simulink model "uas_joystick"  (R2021a)
settings: Solver=VariableStepAuto  StartTime=0.0  StopTime=60  RelTol=1e-3
undefined symbols (not defined in the file or in its folder): Angular, Linear
libraries: robotlib x2, vrlib x1
settings Model: EnablePacing=on  Creator=dwuth  LastModifiedBy=dwuth

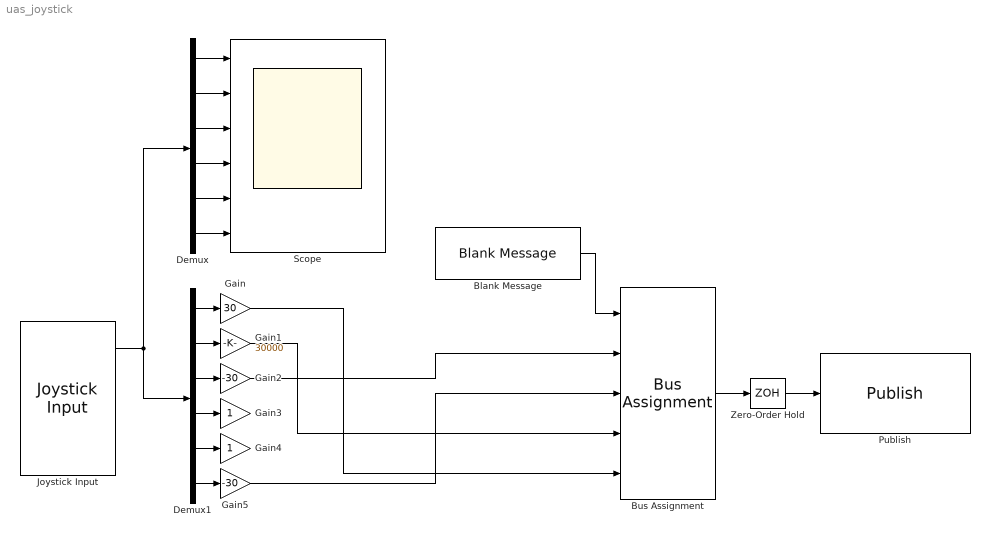
== system uas_joystick ==
  Blank Message : robotlib/Blank Message  messageClass=Message  entityType=geometry_msgs/Twist  messageType=geometry_msgs/Twist  SampleTime=inf  legacyBusStruct=off
  Bus Assignment : BusAssignment  AssignedSignals=Linear.X,Linear.Y,Linear.Z,Angular.Z
  Demux : Demux  Outputs=6
  Demux1 : Demux  Outputs=6
  Gain : Gain  Gain=30
  Gain1 : Gain  Gain=30000
  Gain2 : Gain  Gain=-30
  Gain3 : Gain
  Gain4 : Gain
  Gain5 : Gain  Gain=-30
  Joystick Input : vrlib/Joystick Input  joyid=1  adjustports=on  forcefeed=off
  Publish : robotlib/Publish  topicSource=Specify your own  topic=/crazyflie/cmd_vel  messageType=geometry_msgs/Twist  legacyBusStruct=off  messageQueueLength=1
  Scope : Scope  NumInputPorts=6
  Zero-Order Hold : ZeroOrderHold  SampleTime=25
  wires:
  Demux/1 -> Scope/1
  Demux/2 -> Scope/2
  Demux/3 -> Scope/3
  Demux/4 -> Scope/4
  Demux/5 -> Scope/5
  Demux/6 -> Scope/6
  Joystick Input/1 -> Demux1/1, Demux/1
  Demux1/1 -> Gain/1
  Demux1/2 -> Gain1/1
  Demux1/3 -> Gain2/1
  Demux1/4 -> Gain3/1
  Demux1/5 -> Gain4/1
  Demux1/6 -> Gain5/1
  Blank Message/1 -> Bus Assignment/1
  Zero-Order Hold/1 -> Publish/1
  Bus Assignment/1 -> Zero-Order Hold/1
  Gain2/1 -> Bus Assignment/2
  Gain5/1 -> Bus Assignment/3
  Gain/1 -> Bus Assignment/5
  Gain1/1 -> Bus Assignment/4
